simulink model "gm_iopid_vnl"  (R2021b)
settings: Solver=FixedStepDiscrete  StartTime=0.0  StopTime=100e-3  RelTol=1e-3
libraries: simulink x1, hdlmdlgenlib x1
Description:
  | Symmetric FIR Filter
  | This example shows how to use HDL Coder(TM) to check, generate,
  | and verify HDL for a fixed-point symmetric FIR filter.
settings Model: Creator=The MathWorks, Inc.  LastModifiedBy=Marco Milanesi
settings SolverCC: AlgebraicLoopSolver=TrustRegion  AutoInsertRateTranBlk=on
settings DataIOCC: LimitDataPoints=on  SaveFormat=Array  SaveOutput=off  SignalLogging=off  SaveTime=off  ReturnWorkspaceOutputs=off  SignalLoggingName=logsOut
settings OptimizationCC: BlockReduction=off  BooleanDataType=off  ConditionallyExecuteInputs=off  DefaultParameterBehavior=Inlined  InheritOutputTypeSmallerThanSingle=on  InlineInvariantSignals=on  ExpressionDepthLimit=2147483647  InitFltsAndDblsToZero=on  LifeSpan=inf  BufferReusableBoundary=off
settings DebuggingCC: AlgebraicLoopMsg=error  SaveWithParameterizedLinksMsg=none  UnderspecifiedInitializationDetection=Classic  MergeDetectMultiDrivingBlocksExec=none  CheckExecutionContextPreStartOutputMsg=on  SignalResolutionControl=TryResolveAllWithWarning  InheritedTsInSrcMsg=none  MultiTaskDSMMsg=warning  MultiTaskCondExecSysMsg=none  SingleTaskRateTransMsg=error  IntegerOverflowMsg=none  ParameterPrecisionLossMsg=none  FcnCallInpInsideContextMsg=warning  BusObjectLabelMismatch=none  StateNameClashWarn=warning  SFUnexpectedBacktrackingDiag=warning  SFNoUnconditionalDefaultTransitionDiag=warning  SFExecutionAtInitializationDiag=none  SFMachineParentedDataDiag=warning  IntegerSaturationMsg=none  ArithmeticOperatorsInVariantConditions=warning
settings HardwareCC: ProdBitPerPointer=32  ProdBitPerSizeT=32  ProdBitPerPtrDiffT=32  ProdLargestAtomicFloat=None  ProdIntDivRoundTo=Undefined  ProdEndianess=Unspecified  ProdWordSize=32  ProdHWDeviceType=ASIC/FPGA  TargetUnknown=on  ProdEqTarget=off
settings ModelReferenceCC: PropagateSignalLabelsOutOfModel=off
settings SFSimCC: SimUseLocalCustomCode=off  CustomCodeUndefinedFunction=UseInterfaceOnly
settings RTWCC: RTWUseLocalCustomCode=off
settings CodeAppCC: StateflowObjectComments=on
settings GRTTargetCC: TargetFcnLib=ansi_tfl_tmw.mat  TargetLangStandard=C89/C90 (ANSI)  CombineOutputUpdateFcns=off  GRTInterface=on
settings ConfigComp: CovMetricSettings=dw  CovSaveCumulativeToWorkspaceVar=on  CovSaveSingleToWorkspaceVar=on  CovExternalEMLEnable=off

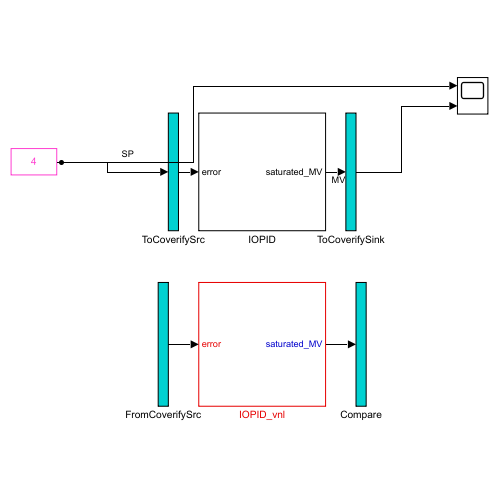
[thumbnail: Simulink's stored preview of the top-level diagram]
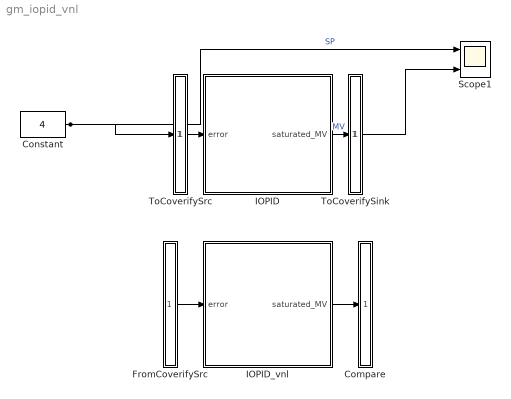
== system gm_iopid_vnl ==
  Compare : Subsystem
      mask Display: disp('')
  Constant : Constant  Value=4  OutDataTypeStr=fixdt(1,32,0)
  FromCoverifySrc : Subsystem
      mask Display: disp('')
  IOPID : Subsystem
  IOPID_vnl : Subsystem
  Scope1 : Scope  NumInputPorts=2
  ToCoverifySink : Subsystem
      mask Display: disp('')
  ToCoverifySrc : Subsystem
      mask Display: disp('')
  wires:
  Constant/1 -> Scope1/1, ToCoverifySrc/1(in1)  "SP"
  ToCoverifySrc/1(out1) -> IOPID/1(error)
  IOPID/1(saturated_MV) -> ToCoverifySink/1(in1)  "MV"
  ToCoverifySink/1(out1) -> Scope1/2
  FromCoverifySrc/1(out1) -> IOPID_vnl/1(error)
  IOPID_vnl/1(saturated_MV) -> Compare/1(in1)

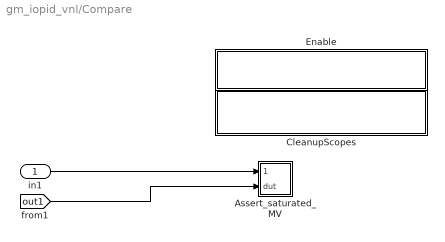
== system gm_iopid_vnl/Compare ==
  in1 : Inport
  Assert_saturated_MV : Subsystem
  CleanupScopes : Subsystem
      settings: OpenFcn=|
      | blkName = gcb; %self block
      | idx = regexp(blkName, '/CleanupScopes$', 'once');
      | blkParent = blkName(1:idx-1);
      | blks=find_system(blkParent, 'LookUnderMasks', 'all','blocktype', 'Scope');
      | for itr = 1:length(blks)
      | 	 hScopeCfg = get_param(blks{itr},'ScopeConfiguration');
      | 	 hScopeCfg.Visible = ~ hScopeCfg.Visible;
      | end
      | drawnow;
      mask Display: fprintf(message('hdlcoder:cosim:vnl_dblclick').getString());
  Enable : Subsystem
      settings: OpenFcn=|
      | blkName = gcb;
      | idx = regexp(blkName, '/Enable$', 'once');
      | blkParent = blkName(1:idx-1);
      | blks=find_system(blkParent, 'LookUnderMasks', 'all','blocktype', 'Assertion');
      | e = get_param(blks{1}, 'Enabled');
      | if strcmp(e, 'on'), f= 'off';, else, f = 'on';, end
      | for ii=1:length(blks), set_param(blks{ii}, 'Enabled', f);, end
      | set_param(gcb, 'MaskDisplay',['fprintf(message(''hdlcoder:cosim:vnl_dblclick_assertions'',','''',upper(e),'''',').getString())']);
      mask Display: fprintf(message('hdlcoder:cosim:vnl_dblclick_assertions','OFF').getString());
  wires:
  in1/1 -> Assert_saturated_MV/1(cosim)
  [out1] -> Assert_saturated_MV/2(dut)

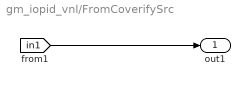
== system gm_iopid_vnl/FromCoverifySrc ==
  out1 : Outport
  wires:
  [in1] -> out1/1

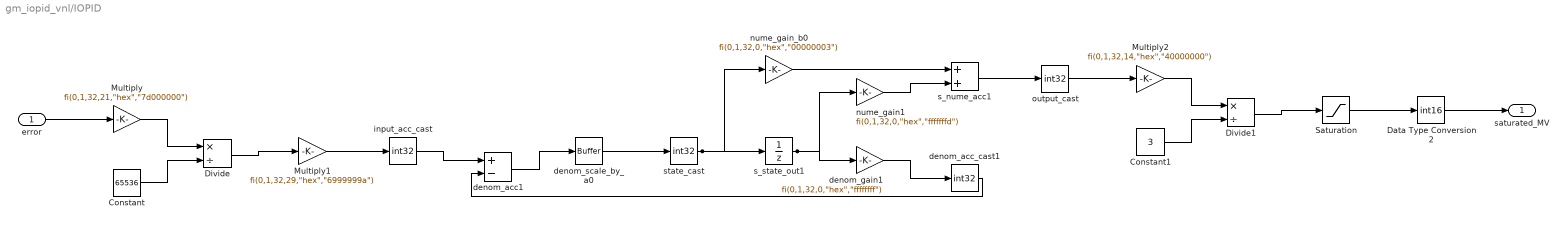
== system gm_iopid_vnl/IOPID ==
  error : Inport  OutDataTypeStr=int32  PortDimensions=1  SampleTime=8e-08
  Constant : Constant  Value=65536  OutDataTypeStr=int32
  Constant1 : Constant  Value=3  OutDataTypeStr=int32
  Data Type Conversion2 : DataTypeConversion  OutDataTypeStr=int16  SampleTime=8e-08
  Divide : Product  Inputs=*/  OutDataTypeStr=int32  RndMeth=Zero  SaturateOnIntegerOverflow=on  SampleTime=8e-08
  Divide1 : Product  Inputs=*/  OutDataTypeStr=int32  RndMeth=Zero  SaturateOnIntegerOverflow=on  SampleTime=8e-08
  Multiply : Gain  Gain="fi(0,1,32,21,\"hex\",\"7d000000\")"  ParamDataTypeStr=fixdt(1, 32, 21)  OutDataTypeStr=int32  SampleTime=8e-08
  Multiply1 : Gain  Gain="fi(0,1,32,29,\"hex\",\"6999999a\")"  ParamDataTypeStr=fixdt(1, 32, 29)  OutDataTypeStr=int32  SampleTime=8e-08
  Multiply2 : Gain  Gain="fi(0,1,32,14,\"hex\",\"40000000\")"  ParamDataTypeStr=fixdt(1, 32, 14)  OutDataTypeStr=int32  SampleTime=8e-08
  Saturation : Saturate  UpperLimit="fi(0,1,32,0,\"hex\",\"000000ff\")"  LowerLimit="fi(0,1,32,0,\"hex\",\"00000000\")"  SampleTime=8e-08  OutDataTypeStr=int32
  denom_acc1 : Sum  Inputs=+-  AccumDataTypeStr=int32  OutDataTypeStr=int32  SampleTime=8e-08
  denom_acc_cast1 : DataTypeConversion  OutDataTypeStr=int32  SampleTime=8e-08
  denom_gain1 : Gain  Gain="fi(0,1,32,0,\"hex\",\"ffffffff\")"  ParamDataTypeStr=fixdt(1, 32, 0)  OutDataTypeStr=int32  SampleTime=8e-08
  denom_scale_by_a0 : hdlmdlgenlib/Buffer
      settings: SourceProductBaseCode=SL
  input_acc_cast : DataTypeConversion  OutDataTypeStr=int32  SampleTime=8e-08
  nume_gain1 : Gain  Gain="fi(0,1,32,0,\"hex\",\"fffffffd\")"  ParamDataTypeStr=fixdt(1, 32, 0)  OutDataTypeStr=int32  SampleTime=8e-08
  nume_gain_b0 : Gain  Gain="fi(0,1,32,0,\"hex\",\"00000003\")"  ParamDataTypeStr=fixdt(1, 32, 0)  OutDataTypeStr=int32  SampleTime=8e-08
  output_cast : DataTypeConversion  OutDataTypeStr=int32  SampleTime=8e-08
  s_nume_acc1 : Sum  OutDataTypeStr=int32  SampleTime=8e-08
  s_state_out1 : UnitDelay  InitialCondition="fi(0,1,32,0,\"hex\",\"00000000\")"  SampleTime=8e-08
  state_cast : DataTypeConversion  OutDataTypeStr=int32  SampleTime=8e-08
  saturated_MV : Outport  OutDataTypeStr=fixdt(1,16,0)  SampleTime=8e-08  VectorParamsAs1DForOutWhenUnconnected=off
  wires:
  output_cast/1 -> Multiply2/1
  s_nume_acc1/1 -> output_cast/1
  nume_gain1/1 -> s_nume_acc1/2
  nume_gain_b0/1 -> s_nume_acc1/1
  denom_gain1/1 -> denom_acc_cast1/1
  s_state_out1/1 -> denom_gain1/1, nume_gain1/1
  state_cast/1 -> s_state_out1/1, nume_gain_b0/1
  denom_scale_by_a0/1 -> state_cast/1
  denom_acc1/1 -> denom_scale_by_a0/1
  denom_acc_cast1/1 -> denom_acc1/2
  input_acc_cast/1 -> denom_acc1/1
  Saturation/1 -> Data Type Conversion2/1
  Multiply2/1 -> Divide1/1
  Multiply1/1 -> input_acc_cast/1
  Multiply/1 -> Divide/1
  Divide1/1 -> Saturation/1
  Divide/1 -> Multiply1/1
  Data Type Conversion2/1 -> saturated_MV/1
  Constant1/1 -> Divide1/2
  Constant/1 -> Divide/2
  error/1 -> Multiply/1

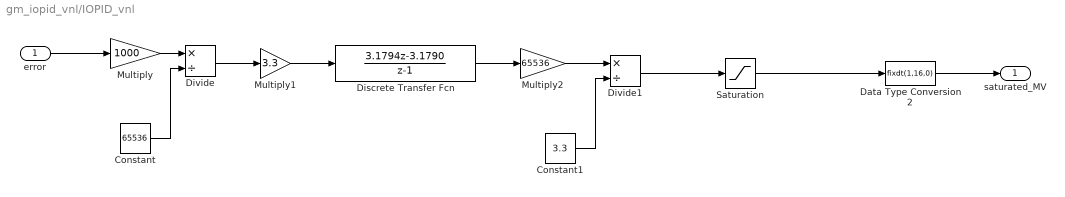
== system gm_iopid_vnl/IOPID_vnl ==
  error : Inport  OutDataTypeStr=fixdt(1,32,0)  SampleTime=80e-9
  Constant : Constant  Value=65536  OutDataTypeStr=fixdt(1,32,0)
  Constant1 : Constant  Value=3.3  OutDataTypeStr=fixdt(1,32,0)
  Data Type Conversion2 : DataTypeConversion  OutDataTypeStr=fixdt(1,16,0)
  Discrete Transfer Fcn : DiscreteTransferFcn  Numerator=[3.1794 -3.1790]  Denominator=[1 -1]  SampleTime=80e-9  NumCoefDataTypeStr=fixdt(1,32,0)  DenCoefDataTypeStr=fixdt(1,32,0)  NumProductDataTypeStr=fixdt(1,32,0)  DenProductDataTypeStr=fixdt(1,32,0)  NumAccumDataTypeStr=fixdt(1,32,0)  DenAccumDataTypeStr=fixdt(1,32,0)  OutDataTypeStr=fixdt(1,32,0)
  Divide : Product  Inputs=*/  OutDataTypeStr=fixdt(1,32,0)  RndMeth=Zero  SaturateOnIntegerOverflow=on
  Divide1 : Product  Inputs=*/  OutDataTypeStr=fixdt(1,32,0)  RndMeth=Zero  SaturateOnIntegerOverflow=on
  Multiply : Gain  Gain=1000  OutDataTypeStr=fixdt(1,32,0)
  Multiply1 : Gain  Gain=3.3  OutDataTypeStr=fixdt(1,32,0)
  Multiply2 : Gain  Gain=65536  OutDataTypeStr=fixdt(1,32,0)
  Saturation : Saturate  UpperLimit=255  LowerLimit=0  OutDataTypeStr=fixdt(1,32,0)
  saturated_MV : Outport  OutDataTypeStr=fixdt(1,16,0)  SampleTime=80e-9  VectorParamsAs1DForOutWhenUnconnected=off
  wires:
  Divide1/1 -> Saturation/1
  Multiply2/1 -> Divide1/1
  Constant1/1 -> Divide1/2
  Discrete Transfer Fcn/1 -> Multiply2/1
  Multiply1/1 -> Discrete Transfer Fcn/1
  Divide/1 -> Multiply1/1
  Constant/1 -> Divide/2
  Multiply/1 -> Divide/1
  error/1 -> Multiply/1
  Saturation/1 -> Data Type Conversion2/1
  Data Type Conversion2/1 -> saturated_MV/1

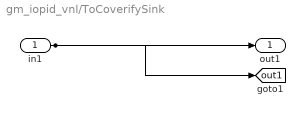
== system gm_iopid_vnl/ToCoverifySink ==
  in1 : Inport
  out1 : Outport
  tag scope: out1=global
  wires:
  in1/1 -> out1/1, [out1]

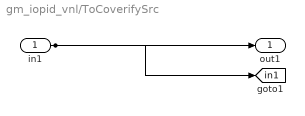
== system gm_iopid_vnl/ToCoverifySrc ==
  in1 : Inport
  out1 : Outport
  tag scope: in1=global
  wires:
  in1/1 -> out1/1, [in1]

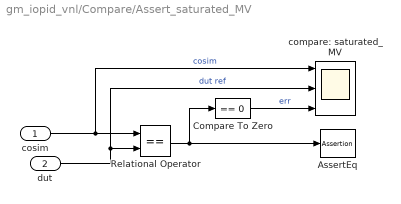
== system gm_iopid_vnl/Compare/Assert_saturated_MV ==
  cosim : Inport
  dut : Inport  Port=2
  AssertEq : Assertion  StopWhenAssertionFail=off
  Compare To Zero : simulink/Logic and Bit Operations/Compare To Zero  relop===  OutDataTypeStr=boolean
  Relational Operator : RelationalOperator  Operator===  OutDataTypeStr=boolean  RndMeth=Nearest
  compare: saturated_MV : Scope  NumInputPorts=3
  wires:
  Compare To Zero/1 -> compare: saturated_MV/3  "err"
  Relational Operator/1 -> Compare To Zero/1, AssertEq/1
  cosim/1 -> compare: saturated_MV/1, Relational Operator/1  "cosim"
  dut/1 -> compare: saturated_MV/2, Relational Operator/2  "dut ref"

== system gm_iopid_vnl/Compare/CleanupScopes ==

== system gm_iopid_vnl/Compare/Enable ==
